simulink model "MyModel_Open_v2"  (R2018b)
settings: Solver=ode23tb  StartTime=0.0  StopTime=0.3  MaxStep=1e-6  RelTol=1e-4
InitFcn:
  | Udc1 = 200;
  | Udc2 = 200;
  | tpwm = 1e-4;
  | ratio = Udc1/Udc2;
  | Td = 2e-6;
  | Kp_current = 3;
  | Ki_current = 120;
libraries: powerlib x31, powerlib_meascontrol x24, powerlib_extras x5, simulink_extras x2, simulink x2
(part 2 of 2)

== matlab function MyModel_Open_v2/SVPWM1/Embedded MATLAB Function1 ==
  data: N input; t1 output; Ualpha input; Ubeta input; Tpwm input; t2 output; t3 output; t4 output; t0 output; udc input; Ux input; Uy input; t1cp output; t2cp output; t3cp output; t4cp output
function [t1, t2, t3, t4, t0, t1cp, t2cp, t3cp, t4cp] = fcn(N, Ualpha, Ubeta, Tpwm, udc, Ux,Uy)

m=sqrt(3)/2+1/2*1i;

%等幅clarke反变换
ab44=1/3*udc*[1,m^4,m^8,m,m^5,m^9]*[1;0;0;1;0;0];
xy44=1/3*udc*[1,m^8,m^4,m^5,m,m^9]*[1;0;0;1;0;0];

ab64=1/3*udc*[1,m^4,m^8,m,m^5,m^9]*[1;1;0;1;0;0];
xy64=1/3*udc*[1,m^8,m^4,m^5,m,m^9]*[1;1;0;1;0;0];
        
ab66=1/3*udc*[1,m^4,m^8,m,m^5,m^9]*[1;1;0;1;1;0];
xy66=1/3*udc*[1,m^8,m^4,m^5,m,m^9]*[1;1;0;1;1;0];

ab26=1/3*udc*[1,m^4,m^8,m,m^5,m^9]*[0;1;0;1;1;0];
xy26=1/3*udc*[1,m^8,m^4,m^5,m,m^9]*[0;1;0;1;1;0];

ab22=1/3*udc*[1,m^4,m^8,m,m^5,m^9]*[0;1;0;0;1;0];
xy22=1/3*udc*[1,m^8,m^4,m^5,m,m^9]*[0;1;0;0;1;0];

ab32=1/3*udc*[1,m^4,m^8,m,m^5,m^9]*[0;1;1;0;1;0];
xy32=1/3*udc*[1,m^8,m^4,m^5,m,m^9]*[0;1;1;0;1;0];

ab33=1/3*udc*[1,m^4,m^8,m,m^5,m^9]*[0;1;1;0;1;1];
xy33=1/3*udc*[1,m^8,m^4,m^5,m,m^9]*[0;1;1;0;1;1];

ab13=1/3*udc*[1,m^4,m^8,m,m^5,m^9]*[0;0;1;0;1;1];
xy13=1/3*udc*[1,m^8,m^4,m^5,m,m^9]*[0;0;1;0;1;1];

ab11=1/3*udc*[1,m^4,m^8,m,m^5,m^9]*[0;0;1;0;0;1];
xy11=1/3*udc*[1,m^8,m^4,m^5,m,m^9]*[0;0;1;0;0;1];

ab51=1/3*udc*[1,m^4,m^8,m,m^5,m^9]*[1;0;1;0;0;1];
xy51=1/3*udc*[1,m^8,m^4,m^5,m,m^9]*[1;0;1;0;0;1];

ab55=1/3*udc*[1,m^4,m^8,m,m^5,m^9]*[1;0;1;1;0;1];
xy55=1/3*udc*[1,m^8,m^4,m^5,m,m^9]*[1;0;1;1;0;1];

ab45=1/3*udc*[1,m^4,m^8,m,m^5,m^9]*[1;0;0;1;0;1];
xy45=1/3*udc*[1,m^8,m^4,m^5,m,m^9]*[1;0;0;1;0;1];

switch N
    case 1
        X=[real(ab55),real(ab45),real(ab44),real(ab64);
           imag(ab55),imag(ab45),imag(ab44),imag(ab64);
           real(xy55),real(xy45),real(xy44),real(xy64);
           imag(xy55),imag(xy45),imag(xy44),imag(xy64)];

    case 2
        X=[real(ab45),real(ab44),real(ab64),real(ab66);
           imag(ab45),imag(ab44),imag(ab64),imag(ab66);
           real(xy45),real(xy44),real(xy64),real(xy66);
           imag(xy45),imag(xy44),imag(xy64),imag(xy66)];

    case 3
        X=[real(ab44),real(ab64),real(ab66),real(ab26);
           imag(ab44),imag(ab64),imag(ab66),imag(ab26);
           real(xy44),real(xy64),real(xy66),real(xy26);
           imag(xy44),imag(xy64),imag(xy66),imag(xy26)];

    case 4
        X=[real(ab64),real(ab66),real(ab26),real(ab22);
           imag(ab64),imag(ab66),imag(ab26),imag(ab22);
           real(xy64),real(xy66),real(xy26),real(xy22);
           imag(xy64),imag(xy66),imag(xy26),imag(xy22)];

    case 5
        X=[real(ab66),real(ab26),real(ab22),real(ab32);
           imag(ab66),imag(ab26),imag(ab22),imag(ab32);
           real(xy66),real(xy26),real(xy22),real(xy32);
           imag(xy66),imag(xy26),imag(xy22),imag(xy32)];

    case 6
        X=[real(ab26),real(ab22),real(ab32),real(ab33);
           imag(ab26),imag(ab22),imag(ab32),imag(ab33);
           real(xy26),real(xy22),real(xy32),real(xy33);
           imag(xy26),imag(xy22),imag(xy32),imag(xy33)];

    case 7
        X=[real(ab22),real(ab32),real(ab33),real(ab13);
           imag(ab22),imag(ab32),imag(ab33),imag(ab13);
           real(xy22),real(xy32),real(xy33),real(xy13);
           imag(xy22),imag(xy32),imag(xy33),imag(xy13)];

    case 8
        X=[real(ab32),real(ab33),real(ab13),real(ab11);
           imag(ab32),imag(ab33),imag(ab13),imag(ab11);
           real(xy32),real(xy33),real(xy13),real(xy11);
           imag(xy32),imag(xy33),imag(xy13),imag(xy11)];

    case 9
        X=[real(ab33),real(ab13),real(ab11),real(ab51);
           imag(ab33),imag(ab13),imag(ab11),imag(ab51);
           real(xy33),real(xy13),real(xy11),real(xy51);
           imag(xy33),imag(xy13),imag(xy11),imag(xy51)];

    case 10
        X=[real(ab13),real(ab11),real(ab51),real(ab55);
           imag(ab13),imag(ab11),imag(ab51),imag(ab55);
           real(xy13),real(xy11),real(xy51),real(xy55);
           imag(xy13),imag(xy11),imag(xy51),imag(xy55)];

    case 11
        X=[real(ab11),real(ab51),real(ab55),real(ab45);
           imag(ab11),imag(ab51),imag(ab55),imag(ab45);
           real(xy11),real(xy51),real(xy55),real(xy45);
           imag(xy11),imag(xy51),imag(xy55),imag(xy45)];

    case 12
        X=[real(ab51),real(ab55),real(ab45),real(ab44);
           imag(ab51),imag(ab55),imag(ab45),imag(ab44);
           real(xy51),real(xy55),real(xy45),real(xy44);
           imag(xy51),imag(xy55),imag(xy45),imag(xy44)];

    otherwise
        X=[0,0,0,0;
           0,0,0,0;
           0,0,0,0;
           0,0,0,0];

end
Y=[Ualpha;Ubeta;Ux;Uy]*Tpwm;
T = X \ Y;

% t1=T(1);
% if t1<15e-6
%     t1=15e-6;
% end
% t2=T(2);
% if t2<15e-6
%     t2=15e-6;
% end
% t3=T(3);
% if t3<1e-6
%     t3=1e-6;
% end
% t4=T(4);
% if t4<1e-6
%     t4=1e-6;
% end

t1=T(1);
t2=T(2);
t3=T(3);
t4=T(4);
t1cp = 0;
t2cp = 0;
t3cp = 0;
t4cp = 0;
% if T(1) >= 0
%     t1 = T(1);
% else
%     t1 = 0;
%     t1cp = -T(1);
% end
% if T(2) >= 0
%     t2 = T(2);
% else
%     t2 = 0;
%     t2cp = -T(2);
% end
% if T(3) >= 0
%     t3 = T(3);
% else
%     t3 = 0;
%     t3cp = -T(3);
% end
% if T(4) >= 0
%     t4 = T(4);
% else
%     t4 = 0;
%     t4cp = -T(4);
% end

Tsum=t1+t2+t3+t4;
if Tsum>Tpwm
    t1=t1*Tpwm/Tsum;
    t2=t2*Tpwm/Tsum;
    t3=t3*Tpwm/Tsum;
    t4=t4*Tpwm/Tsum;
end
t0=Tpwm-t1-t2-t3-t4;
end

== matlab function MyModel_Open_v2/SVPWM1/rest of others ==
  data: N input; T1 input; T2 input; T3 input; T4 input; T0 input; a1 output; a2 output; b1 output; b2 output; c1 output; c2 output; d1 output; d2 output; e1 output; e2 output; f1 output; f2 output; t1cp input; t2cp input; t3cp input; t4cp input
function [a1,a2,b1,b2,c1,c2,d1,d2,e1,e2,f1,f2] = fcn(N,T1,T2,T3,T4,T0,t1cp,t2cp,t3cp,t4cp)

%#xsxx
Ta=T0/4;
Tb=Ta+T2;
Tc=Tb+T1;
Td=Tc+T0/2;
Te=Td+T4;
Tf=Te+T3;

Ta1=T0/4;
Tb1=Ta1+T1;
Tc1=Tb1+T2;
Td1=Tc1+T0/2;
Te1=Td1+T3;
Tf1=Te1+T4;

%a1:phase A CMPA
%a2:phase A CMPB

a1 = 0;
a2 = 0;
b1 = 0;
b2 = 0;
c1 = 0;
c2 = 0;
d1 = 0;
d2 = 0;
e1 = 0;
e2 = 0;
f1 = 0;
f2 = 0;

if N==1
    a1=Ta;%TIme of "00" voltage vector 
    a2=Tf;%TIme of "48" voltage vector 
    d1=Ta;
    d2=Tf;
    b1=Tc;%TIme of "51" voltage vector 
    b2=Te + t1cp + t2cp + t3cp;%TIme of "56" voltage vector 
    e1=Tc;
    e2=Td + t1cp +t2cp +t3cp + t4cp;
    c1=Tb;%TIme of "49" voltage vector 
    c2=Td + t2cp + t3cp + t4cp;%TIme of "63" voltage vector 
    f1=Ta;
    f2=Td + t3cp + t4cp;
elseif N==2
    a1=Ta;
    a2=Tf;
    d1=Ta;
    d2=Tf;
    b1=Tc;
    b2=Tf + t1cp + t2cp;
    e1=Tc;
    e2=Te + t1cp + t2cp + t3cp;
    c1=Tc;
    c2=Td + t1cp + t2cp + t3cp + t4cp;
    f1=Tb;
    f2=Td + t2cp + t3cp + t4cp;
elseif N==3
    a1=Ta1;
    a2=Te1 + t4cp;
    d1=Ta1;
    d2=Tf1;
    b1=Tb1;
    b2=Tf1 + t1cp;
    e1=Tc1;
    e2=Tf1 + t1cp + t2cp;
    c1=Tc1;
    c2=Td1 + t1cp + t2cp + t3cp + t4cp;
    f1=Tc1;
    f2=Td1 + t1cp + t2cp + t3cp + t4cp;
elseif N==4
    a1=Ta1;
    a2=Td1 + t3cp + t4cp;
    d1=Ta1;
    d2=Te1 + t4cp;
    b1=Ta1;
    b2=Tf1;
    e1=Tb1;
    e2=Tf1 + t1cp;
    c1=Tc1;
    c2=Td1 + t1cp + t2cp + t3cp + t4cp;
    f1=Tc1;
    f2=Td1 + t1cp + t2cp + t3cp + t4cp;
elseif N==5
    a1=Tb;
    a2=Td + t2cp + t3cp + t4cp;
    d1=Ta;
    d2=Td + t3cp + t4cp;
    b1=Ta;
    b2=Tf;
    e1=Ta;
    e2=Tf;
    c1=Tc;
    c2=Te + t1cp + t2cp + t3cp;
    f1=Tc;
    f2=Td + t1cp + t2cp + t3cp + t4cp;
elseif N==6
    a1=Tc;
    a2=Td + t1cp + t2cp + t3cp + t4cp;
    d1=Tb;
    d2=Td + t2cp + t3cp + t4cp;
    b1=Ta;
    b2=Tf;
    e1=Ta;
    e2=Tf;
    c1=Tc;
    c2=Tf + t1cp + t2cp;
    f1=Tc;
    f2=Te + t1cp + t2cp + t3cp;
elseif N==7
    a1=Tc1;
    a2=Td1 + t1cp + t2cp + t3cp + t4cp;
    d1=Tc1;
    d2=Td1 + t1cp + t2cp + t3cp + t4cp;
    b1=Ta1;
    b2=Te1 + t4cp;
    e1=Ta1;
    e2=Tf1;
    c1=Tb1;
    c2=Tf1 + t1cp;
    f1=Tc1;
    f2=Tf1 + t1cp + t2cp;
elseif N==8
    a1=Tc1;
    a2=Td1 + t1cp + t2cp + t3cp + t4cp;
    d1=Tc1;
    d2=Td1 + t1cp + t2cp + t3cp + t4cp;
    b1=Ta1;
    b2=Td1 + t3cp + t4cp;
    e1=Ta1;
    e2=Te1 + t4cp;
    c1=Ta1;
    c2=Tf1;
    f1=Tb1;
    f2=Tf1 + t1cp;
elseif N==9
    a1=Tc;
    a2=Te + t1cp + t2cp + t3cp;
    d1=Tc;
    d2=Td + t1cp + t2cp + t3cp + t4cp;
    b1=Tb;
    b2=Td + t2cp + t3cp + t4cp;
    e1=Ta;
    e2=Td + t3cp + t4cp;
    c1=Ta;
    c2=Tf;
    f1=Ta;
    f2=Tf;
elseif N==10
    a1=Tc;
    a2=Tf + t1cp + t2cp;
    d1=Tc;
    d2=Te + t1cp + t2cp + t3cp;
    b1=Tc;
    b2=Td + t1cp + t2cp + t3cp + t4cp;
    e1=Tb;
    e2=Td + t2cp + t3cp + t4cp;
    c1=Ta;
    c2=Tf;
    f1=Ta;
    f2=Tf;
elseif N==11
    a1=Tb1;
    a2=Tf1 + t1cp;
    d1=Tc1;
    d2=Tf1 + t1cp + t2cp;
    b1=Tc1;
    b2=Td1 + t1cp + t2cp + t3cp + t4cp;
    e1=Tc1;
    e2=Td1 + t1cp + t2cp + t3cp + t4cp;
    c1=Ta1;
    c2=Te1 + t4cp;
    f1=Ta1;
    f2=Tf1;
elseif N==12
    a1=Ta1;
    a2=Tf1;
    d1=Tb1;
    d2=Tf1 + t1cp;
    b1=Tc1;
    b2=Td1 + t1cp + t2cp + t3cp + t4cp;
    e1=Tc1;
    e2=Td1 + t1cp + t2cp + t3cp + t4cp;
    c1=Ta1;
    c2=Td1 + t3cp + t4cp;
    f1=Ta1;
    f2=Te1 + t4cp;
end
